simulink model "carga_new"  (R2018a)
settings: Solver=ode8  StartTime=0.0  StopTime=10.0  FixedStep=0.0001  RelTol=1e-3
InitFcn:
  | SimulinkInit_linea_transmision
values from neighbouring files (symbols this model uses):
  Cl = 20000e-6    (= 0.02)    [SimulinkInit_linea_transmision.m]
  L = 5.2    [SimulinkInit_linea_transmision.m]
  R = 10    [SimulinkInit_linea_transmision.m]
  RL = 10    [SimulinkInit_linea_transmision.m]
libraries: powerlib_meascontrol x1
settings Model: Creator=MarioAndres  LastModifiedBy=MarioAndres
settings OptimizationCC: DefaultParameterBehavior=Inlined  EnhancedBackFolding=on  PassReuseOutputArgsAs=Individual arguments  OptimizeBlockOrder=speed  DifferentSizesBufferReuse=on  OptimizationCustomize=off
settings DebuggingCC: ParameterTunabilityLossMsg=error
settings SFSimCC: MATLABDynamicMemAlloc=off
settings RTWCC: SystemTargetFile=ert.tlc  TemplateMakefile=ert_default_tmf  GenerateReport=on  IncludeHyperlinkInReport=on  LaunchReport=on  GenerateTraceInfo=on  GenerateTraceReport=on  GenerateTraceReportSl=on  GenerateTraceReportSf=on  GenerateTraceReportEml=on
settings CodeAppCC: ForceParamTrailComments=on  IgnoreCustomStorageClasses=off  OperatorAnnotations=on  SimulinkDataObjDesc=on  SFDataObjDesc=on  InsertBlockDesc=on
settings ERTTargetCC: TargetLangStandard=C99 (ISO)  GenerateSampleERTMain=on  SupportContinuousTime=on  InlinedParameterPlacement=NonHierarchical  ERTCustomFileTemplate=example_file_process.tlc

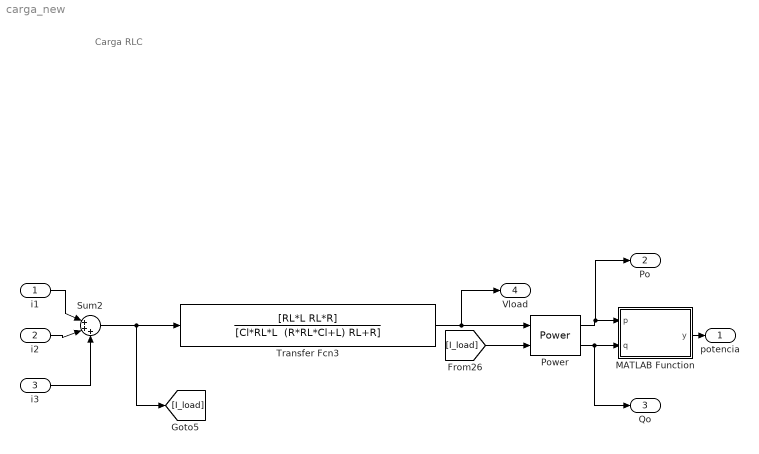
== system carga_new ==
  note: Carga RLC
  i1 : Inport
  i2 : Inport  Port=2
  i3 : Inport  Port=3
  MATLAB Function : MATLAB Function  TreatAsAtomicUnit=on
  Power : powerlib_meascontrol/Measurements/Power  Freq=60  Vinit=[1, 0]  Iinit=[1, 0]  Ts=0
      settings: SourceProductName=Simscape Power Systems
  Sum2 : Sum  Inputs=|+++
  Transfer Fcn3 : TransferFcn  Numerator=[RL*L RL*R]  Denominator="[Cl*RL*L  (R*RL*Cl+L) RL+R]"
  potencia : Outport
  Po : Outport  Port=2
  Qo : Outport  Port=3
  Vload : Outport  Port=4
  wires:
  Sum2/1 -> [I_load], Transfer Fcn3/1
  [I_load] -> Power/2
  Transfer Fcn3/1 -> Vload/1, Power/1
  Power/2 -> Qo/1, MATLAB Function/2(q)
  Power/1 -> Po/1, MATLAB Function/1(p)
  i1/1 -> Sum2/1
  i2/1 -> Sum2/2
  i3/1 -> Sum2/3
  MATLAB Function/1(y) -> potencia/1

== matlab function carga_new/MATLAB Function ==
  data: p input; y output; q input
function y = fcn(p,q)

y = sqrt(p^2+q^2);
